simulink model "zad8simulink"  (R2023a)
settings: Solver=VariableStepAuto  StartTime=0.0  StopTime=10  RelTol=1e-3
values from neighbouring files (symbols this model uses):
  Gz = c2d(Gs,T,'zoh')    [zad1.m]
  Kpor = acker(A,B,bieguny)    [zad4.m]
  Lpor = acker(A',C',[b_obsv,b_obsv,b_obsv])'    [zad6.m]
  T = 0.5    [zad1.m]    (also in zad4.mat)
settings Model: Creator=pkutyl  LastModifiedBy=pkutyl

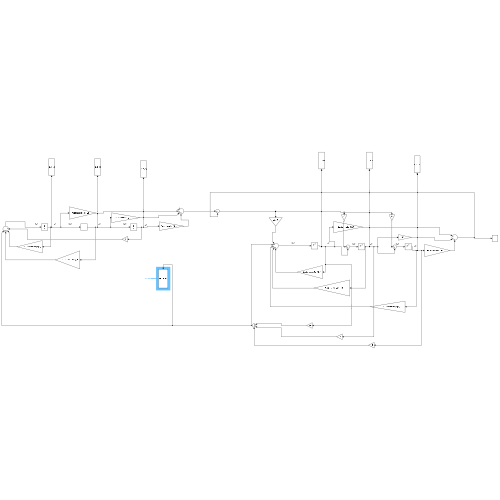
[thumbnail: Simulink's stored preview of the top-level diagram]
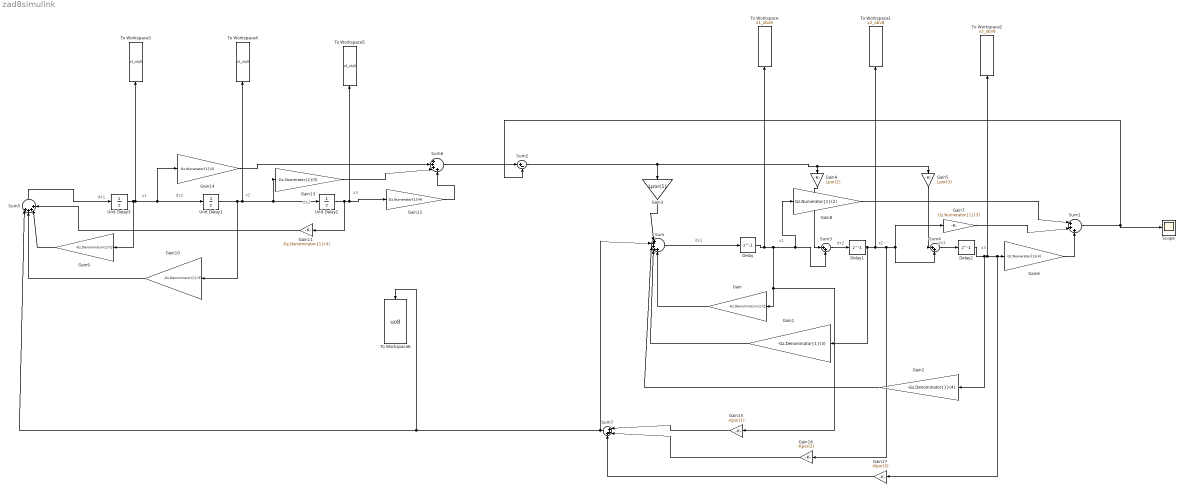
== system zad8simulink ==
  note: dx2
  note: dx1
  note: x1
  note: dx3
  note: x2
  note: dx1
  note: x2
  note: x3
  note: x1
  note: dx2
  note: dx3
  note: x3
  Delay : Delay  DelayLength=1  InitialCondition=0  SampleTime=T
  Delay1 : Delay  DelayLength=1  InitialCondition=0  SampleTime=T
  Delay2 : Delay  DelayLength=1  InitialCondition=0  SampleTime=T
  Gain : Gain  Gain=-Gz.Denominator{1}(2)
  Gain1 : Gain  Gain=-Gz.Denominator{1}(3)
  Gain10 : Gain  Gain=-Gz.Denominator{1}(3)
  Gain11 : Gain  Gain=-Gz.Denominator{1}(4)
  Gain12 : Gain  Gain=Gz.Numerator{1}(4)
  Gain13 : Gain  Gain=Gz.Numerator{1}(3)
  Gain14 : Gain  Gain=Gz.Numerator{1}(2)
  Gain15 : Gain  Gain=-Kpor(1)
  Gain16 : Gain  Gain=-Kpor(2)
  Gain17 : Gain  Gain=-Kpor(3)
  Gain2 : Gain  Gain=-Gz.Denominator{1}(4)
  Gain3 : Gain  Gain=Lpor(1)
  Gain4 : Gain  Gain=Lpor(2)
  Gain5 : Gain  Gain=Lpor(3)
  Gain6 : Gain  Gain=Gz.Numerator{1}(4)
  Gain7 : Gain  Gain=Gz.Numerator{1}(3)
  Gain8 : Gain  Gain=Gz.Numerator{1}(2)
  Gain9 : Gain  Gain=-Gz.Denominator{1}(2)
  Scope : Scope
  Sum : Sum  Inputs=|+++++
  Sum1 : Sum  Inputs=|+++
  Sum2 : Sum  Inputs=|+-
  Sum3 : Sum  Inputs=|++
  Sum4 : Sum  Inputs=|++
  Sum5 : Sum  Inputs=|++++
  Sum6 : Sum  Inputs=|++++
  Sum7 : Sum  Inputs=|+++
  To Workspace : ToWorkspace  VariableName=x1_obv8  SaveFormat=Structure With Time  SampleTime=-1
  To Workspace1 : ToWorkspace  VariableName=x2_obv8  SaveFormat=Structure With Time  SampleTime=-1
  To Workspace2 : ToWorkspace  VariableName=x3_obv8  SaveFormat=Structure With Time  SampleTime=-1
  To Workspace3 : ToWorkspace  VariableName=x1_obj8  SaveFormat=Structure With Time  SampleTime=-1
  To Workspace4 : ToWorkspace  VariableName=x2_obj8  SaveFormat=Structure With Time  SampleTime=-1
  To Workspace5 : ToWorkspace  VariableName=x3_obj8  SaveFormat=Structure With Time  SampleTime=-1
  To Workspace6 : ToWorkspace  VariableName=uo8  SaveFormat=Structure With Time  SampleTime=-1
  Unit Delay1 : UnitDelay  InitialCondition=1  SampleTime=T  HasFrameUpgradeWarning=on
  Unit Delay2 : UnitDelay  InitialCondition=-1  SampleTime=T  HasFrameUpgradeWarning=on
  Unit Delay3 : UnitDelay  InitialCondition=2  SampleTime=T  HasFrameUpgradeWarning=on
  wires:
  Sum5/1 -> Unit Delay3/1
  Delay2/1 -> To Workspace2/1, Gain17/1, Gain6/1, Gain2/1
  Delay/1 -> To Workspace/1, Gain15/1, Gain/1, Sum3/2, Gain8/1
  Sum4/1 -> Delay2/1
  Gain10/1 -> Sum5/2
  Delay1/1 -> To Workspace1/1, Gain16/1, Gain7/1, Sum4/2, Gain1/1
  Gain1/1 -> Sum/4
  Sum6/1 -> Sum2/1
  Sum/1 -> Delay/1
  Gain12/1 -> Sum6/4
  Gain9/1 -> Sum5/3
  Gain8/1 -> Sum1/1
  Unit Delay1/1 -> Gain10/1, Gain13/1, Unit Delay2/1, To Workspace4/1
  Unit Delay2/1 -> Gain12/1, To Workspace5/1, Gain11/1
  Gain5/1 -> Sum4/1
  Gain3/1 -> Sum/1
  Sum1/1 -> Sum2/2, Scope/1
  Gain6/1 -> Sum1/3
  Gain7/1 -> Sum1/2
  Gain/1 -> Sum/5
  Sum2/1 -> Gain5/1, Gain4/1, Gain3/1
  Gain2/1 -> Sum/3
  Gain13/1 -> Sum6/3
  Sum3/1 -> Delay1/1
  Unit Delay3/1 -> Gain9/1, Unit Delay1/1, Gain14/1, To Workspace3/1
  Gain4/1 -> Sum3/1
  Gain11/1 -> Sum5/4
  Gain14/1 -> Sum6/2
  Gain15/1 -> Sum7/1
  Gain16/1 -> Sum7/2
  Gain17/1 -> Sum7/3
  Sum7/1 -> Sum/2, To Workspace6/1, Sum5/1
